simulink model "es1_sim"  (R2023b)
settings: Solver=VariableStepAuto  StartTime=0.0  StopTime=10.0  RelTol=1e-3
values from neighbouring files (symbols this model uses):
  A = [-1 5 ... (first row only)    [es1_mio.m]
  B = [1;0]    [es1_mio.m]
  C = [1 5]    [es1_mio.m]
settings Model: Creator=stefa  LastModifiedBy=stefa

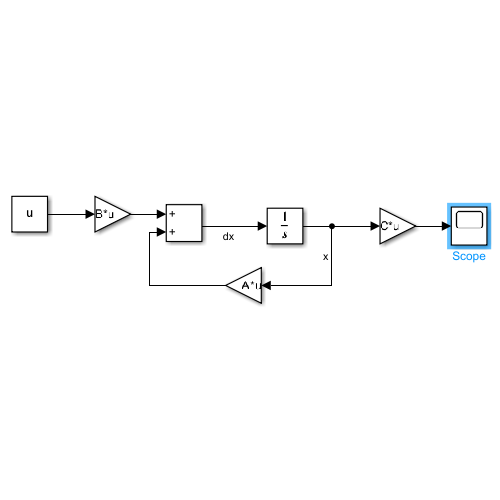
[thumbnail: Simulink's stored preview of the top-level diagram]
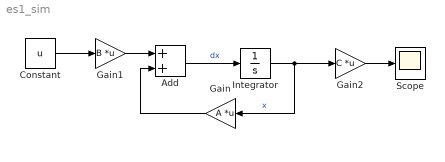
== system es1_sim ==
  Add : Sum
  Constant : Constant  Value=u
  Gain : Gain  Gain=A  Multiplication=Matrix(K*u)
  Gain1 : Gain  Gain=B  Multiplication=Matrix(K*u)
  Gain2 : Gain  Gain=C  Multiplication=Matrix(K*u)
  Integrator : Integrator
  Scope : Scope
  wires:
  Gain1/1 -> Add/1
  Constant/1 -> Gain1/1
  Add/1 -> Integrator/1  "dx"
  Integrator/1 -> Gain2/1, Gain/1  "x"
  Gain/1 -> Add/2
  Gain2/1 -> Scope/1
